simulink model "SKML"  (R2020a)
settings: Solver=VariableStepAuto  StartTime=0.0  StopTime=10.0  RelTol=1e-3
settings Model: Creator=alfan  LastModifiedBy=alfan

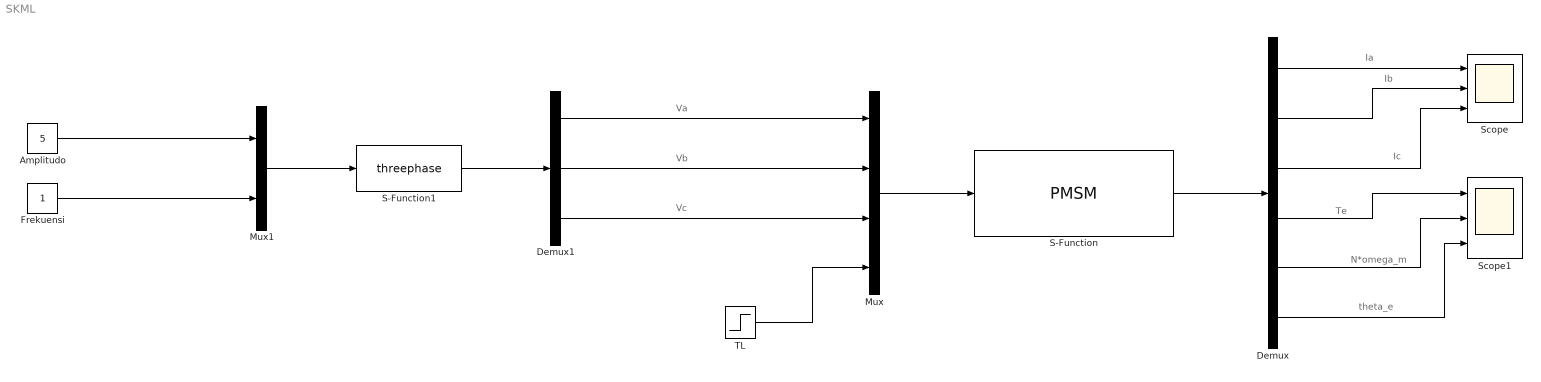
== system SKML ==
  note: Va
  note: theta_e
  note: N*omega_m
  note: Te
  note: Ic
  note: Ib
  note: Ia
  note: Vb
  note: Vc
  Amplitudo : Constant  Value=5
  Demux : Demux  Outputs=6
  Demux1 : Demux  Outputs=3
  Frekuensi : Constant
  Mux : Mux
  Mux1 : Mux  Inputs=2
  S-Function : S-Function  FunctionName=PMSM  SFunctionDeploymentMode=off  EnableBusSupport=off
  S-Function1 : S-Function  FunctionName=threephase  SFunctionDeploymentMode=off  EnableBusSupport=off
  Scope : Scope  NumInputPorts=3
  Scope1 : Scope  NumInputPorts=3
  TL : Step  SampleTime=0
  wires:
  Mux/1 -> S-Function/1
  S-Function/1 -> Demux/1
  TL/1 -> Mux/4
  Demux1/3 -> Mux/3
  Demux/1 -> Scope/1
  Demux/2 -> Scope/2
  Demux/3 -> Scope/3
  Demux/4 -> Scope1/1
  Demux/5 -> Scope1/2
  Demux/6 -> Scope1/3
  Demux1/2 -> Mux/2
  Demux1/1 -> Mux/1
  S-Function1/1 -> Demux1/1
  Mux1/1 -> S-Function1/1
  Frekuensi/1 -> Mux1/2
  Amplitudo/1 -> Mux1/1
